simulink subsystem "WiW2025WTSubV2"  (R2024b)
settings: Solver=VariableStepAuto  StartTime=0.0  StopTime=10.0  RelTol=1e-3
values from neighbouring files (symbols this model uses):
  parWT_Init =     [parWT_Init.mat]
undefined symbols (not defined in the file or in its folder): DiscIntNeverNeededParam
settings Model: Creator=jb  LastModifiedBy=jb

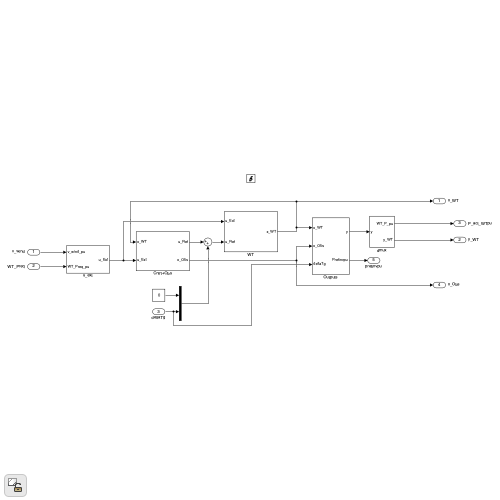
[thumbnail: Simulink's stored preview of the top-level diagram]
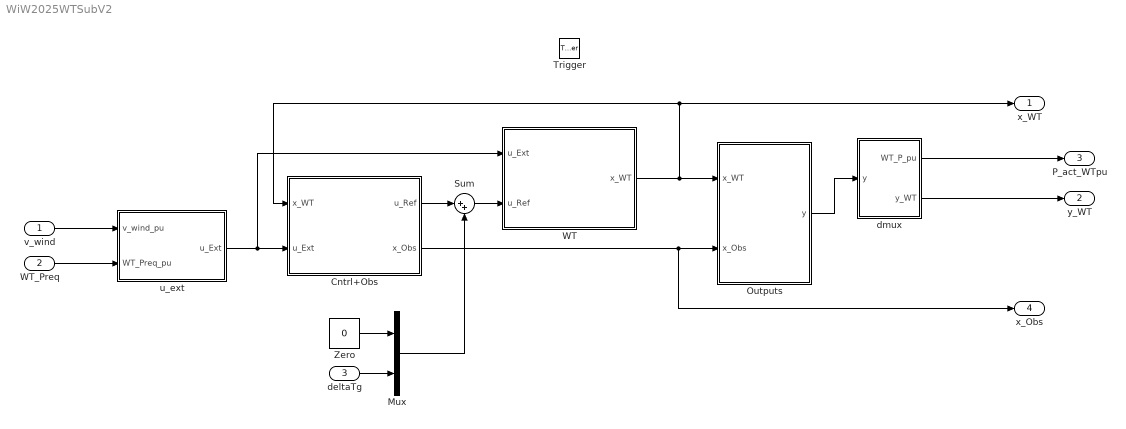
== system WiW2025WTSubV2 ==
  v_wind : Inport
  WT_Preq : Inport  Port=2
  deltaTg : Inport  Port=3
  Trigger : TriggerPort  VariantControl=(inherit)  InitialTriggerSignalState=zero
  Cntrl+Obs : Subsystem
  Mux : Mux  Inputs=2
  Outputs : Subsystem
  Sum : Sum  Inputs=|++
  WT : Subsystem
  Zero : Constant  Value=0  OutDataTypeStr=Inherit: Inherit via back propagation
  dmux : Subsystem
  u_ext : Subsystem
  x_WT : Outport
  y_WT : Outport  Port=2
  P_act_WTpu : Outport  Port=3
  x_Obs : Outport  Port=4
  wires:
  u_ext/1(u_Ext) -> Cntrl+Obs/2(u_Ext), WT/1(u_Ext)
  dmux/2(y_WT) -> y_WT/1
  WT/1(x_WT) -> Outputs/1(x_WT), Cntrl+Obs/1(x_WT), x_WT/1
  v_wind/1 -> u_ext/1(v_wind_pu)
  WT_Preq/1 -> u_ext/2(WT_Preq_pu)
  dmux/1(WT_P_pu) -> P_act_WTpu/1
  Cntrl+Obs/2(x_Obs) -> Outputs/2(x_Obs), x_Obs/1
  Outputs/1(y) -> dmux/1(y)
  Zero/1 -> Mux/1
  deltaTg/1 -> Mux/2
  Cntrl+Obs/1(u_Ref) -> Sum/1
  Sum/1 -> WT/2(u_Ref)
  Mux/1 -> Sum/2

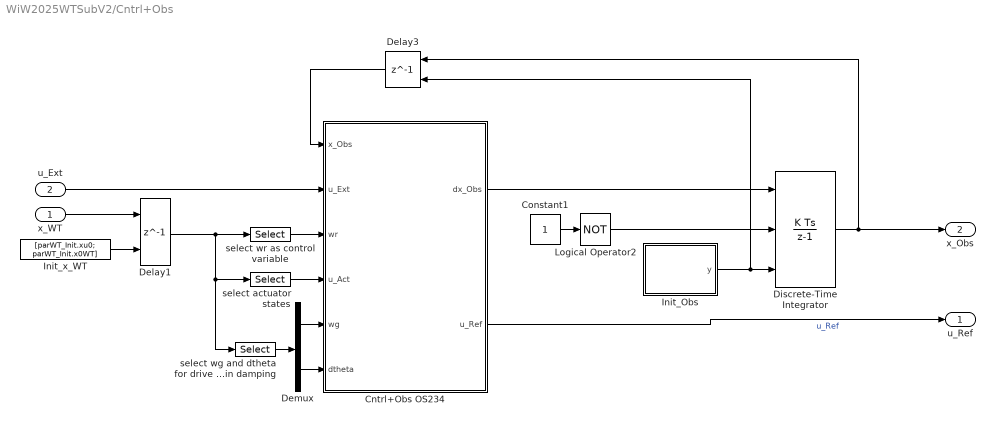
== system WiW2025WTSubV2/Cntrl+Obs ==
  x_WT : Inport  OutDataTypeStr=double  PortDimensions=11
  u_Ext : Inport  Port=2  OutDataTypeStr=double  PortDimensions=2
  Cntrl+Obs OS234 : MATLAB Function  TreatAsAtomicUnit=on
  Constant1 : Constant
  Delay1 : Delay  DelayLength=1  InitialConditionSource=Input port  InitialCondition=0
      settings: InputPortMap=u0,p4
  Delay3 : Delay  DelayLength=1  InitialConditionSource=Input port
      settings: InputPortMap=u0,p4
  Demux : Demux  Outputs=2
  Discrete-Time Integrator : DiscreteIntegrator  ExternalReset=level  InitialConditionSource=external  SampleTime=-1  ICPrevOutput=DiscIntNeverNeededParam  ICPrevScaledInput=DiscIntNeverNeededParam
  Init_Obs : MATLAB Function  TreatAsAtomicUnit=on
  Init_x_WT : Constant  Value=[parWT_Init.xu0; parWT_Init.x0WT]  VectorParams1D=off
  Logical Operator2 : Logic  Operator=NOT  AllPortsSameDT=off  OutDataTypeStr=boolean
  select actuator states : Selector  InputPortWidth=11  IndexOptions=Index vector (dialog)  Indices=[1 2]  OutputSizes=1
  select wg and dtheta for drive train damping : Selector  InputPortWidth=11  IndexOptions=Index vector (dialog)  Indices=[10,11]  OutputSizes=1
  select wr as control variable : Selector  InputPortWidth=11  IndexOptions=Index vector (dialog)  Indices=[9]  OutputSizes=1
  u_Ref : Outport  OutDataTypeStr=double  PortDimensions=2
  x_Obs : Outport  Port=2  OutDataTypeStr=double  PortDimensions=2
  wires:
  Demux/2 -> Cntrl+Obs OS234/6(dtheta)
  Demux/1 -> Cntrl+Obs OS234/5(wg)
  select wg and dtheta for drive train damping/1 -> Demux/1
  Logical Operator2/1 -> Discrete-Time Integrator/2
  Discrete-Time Integrator/1 -> x_Obs/1, Delay3/1
  Cntrl+Obs OS234/2(u_Ref) -> u_Ref/1  "u_Ref"
  select actuator states/1 -> Cntrl+Obs OS234/4(u_Act)
  Delay1/1 -> select wr as control variable/1, select actuator states/1, select wg and dtheta for drive train damping/1
  select wr as control variable/1 -> Cntrl+Obs OS234/3(wr)
  u_Ext/1 -> Cntrl+Obs OS234/2(u_Ext)
  Delay3/1 -> Cntrl+Obs OS234/1(x_Obs)
  Cntrl+Obs OS234/1(dx_Obs) -> Discrete-Time Integrator/1
  Init_x_WT/1 -> Delay1/2
  x_WT/1 -> Delay1/1
  Constant1/1 -> Logical Operator2/1
  Init_Obs/1(y) -> Delay3/2, Discrete-Time Integrator/3

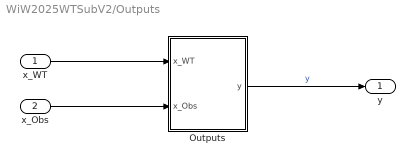
== system WiW2025WTSubV2/Outputs ==
  x_WT : Inport  OutDataTypeStr=double  PortDimensions=11
  x_Obs : Inport  Port=2  OutDataTypeStr=double  PortDimensions=2
  Outputs : MATLAB Function  TreatAsAtomicUnit=on
  y : Outport  OutDataTypeStr=double  PortDimensions=14
  wires:
  Outputs/1(y) -> y/1  "y"
  x_Obs/1 -> Outputs/2(x_Obs)
  x_WT/1 -> Outputs/1(x_WT)

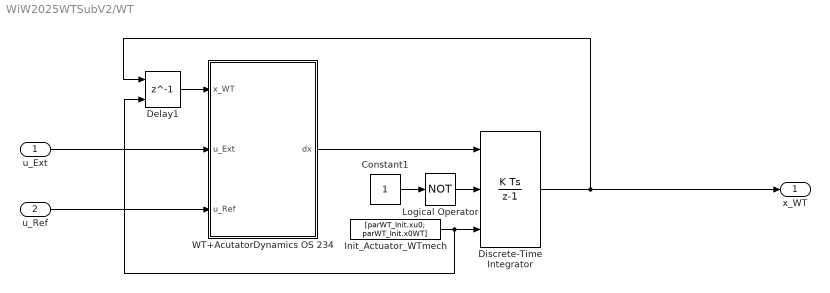
== system WiW2025WTSubV2/WT ==
  u_Ext : Inport  OutDataTypeStr=double  PortDimensions=2
  u_Ref : Inport  Port=2  OutDataTypeStr=double  PortDimensions=2
  Constant1 : Constant
  Delay1 : Delay  DelayLength=1  InitialConditionSource=Input port
      settings: InputPortMap=u0,p4
  Discrete-Time Integrator : DiscreteIntegrator  ExternalReset=level  InitialConditionSource=external  SampleTime=-1  ICPrevOutput=DiscIntNeverNeededParam  ICPrevScaledInput=DiscIntNeverNeededParam
  Init_Actuator_WTmech : Constant  Value=[parWT_Init.xu0; parWT_Init.x0WT]  VectorParams1D=off
  Logical Operator : Logic  Operator=NOT  AllPortsSameDT=off  OutDataTypeStr=boolean
  WT+AcutatorDynamics OS 234 : MATLAB Function  TreatAsAtomicUnit=on
  x_WT : Outport  OutDataTypeStr=double  PortDimensions=11
  wires:
  u_Ext/1 -> WT+AcutatorDynamics OS 234/2(u_Ext)
  Logical Operator/1 -> Discrete-Time Integrator/2
  Constant1/1 -> Logical Operator/1
  Init_Actuator_WTmech/1 -> Discrete-Time Integrator/3, Delay1/2
  u_Ref/1 -> WT+AcutatorDynamics OS 234/3(u_Ref)
  WT+AcutatorDynamics OS 234/1(dx) -> Discrete-Time Integrator/1
  Discrete-Time Integrator/1 -> x_WT/1, Delay1/1
  Delay1/1 -> WT+AcutatorDynamics OS 234/1(x_WT)

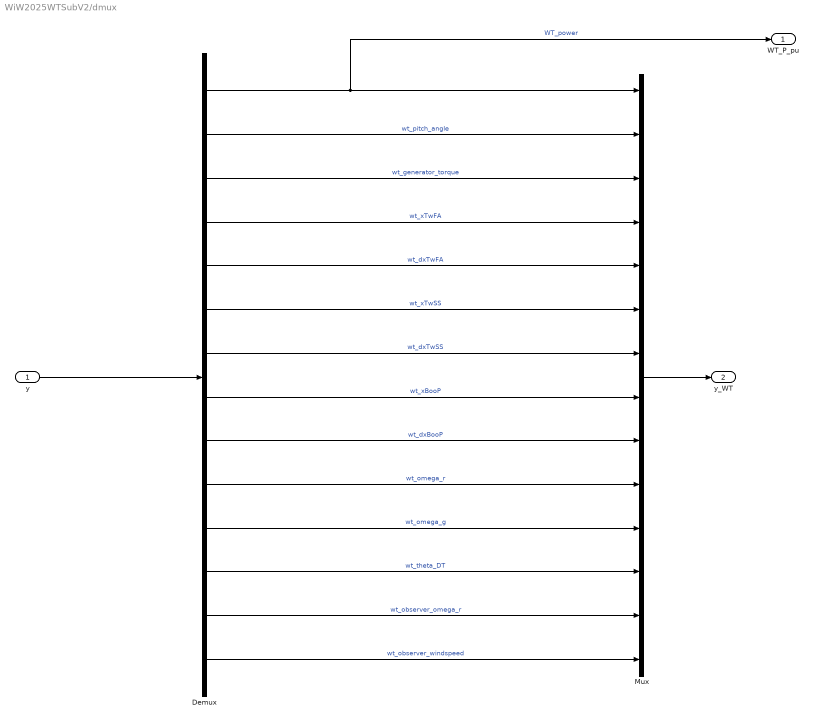
== system WiW2025WTSubV2/dmux ==
  y : Inport  OutDataTypeStr=double  PortDimensions=14
  Demux : Demux  Outputs=14
  Mux : Mux  Inputs=14
  WT_P_pu : Outport  OutDataTypeStr=double  PortDimensions=1
  y_WT : Outport  Port=2  OutDataTypeStr=double  PortDimensions=14
  wires:
  Demux/8 -> Mux/8  "wt_xBooP"
  Demux/5 -> Mux/5  "wt_dxTwFA"
  Demux/9 -> Mux/9  "wt_dxBooP"
  Demux/11 -> Mux/11  "wt_omega_g"
  Demux/12 -> Mux/12  "wt_theta_DT"
  Demux/1 -> WT_P_pu/1, Mux/1  "WT_power"
  Demux/7 -> Mux/7  "wt_dxTwSS"
  Demux/6 -> Mux/6  "wt_xTwSS"
  y/1 -> Demux/1
  Demux/3 -> Mux/3  "wt_generator_torque"
  Demux/14 -> Mux/14  "wt_observer_windspeed"
  Demux/10 -> Mux/10  "wt_omega_r"
  Demux/4 -> Mux/4  "wt_xTwFA"
  Demux/13 -> Mux/13  "wt_observer_omega_r"
  Demux/2 -> Mux/2  "wt_pitch_angle"
  Mux/1 -> y_WT/1

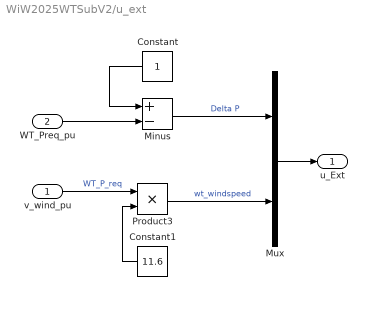
== system WiW2025WTSubV2/u_ext ==
  v_wind_pu : Inport
  WT_Preq_pu : Inport  Port=2
  Constant : Constant
  Constant1 : Constant  Value=11.6
  Minus : Sum  Inputs=+-
  Mux : Mux  Inputs=2
  Product3 : Product
  u_Ext : Outport
  wires:
  v_wind_pu/1 -> Product3/1  "WT_P_req"
  WT_Preq_pu/1 -> Minus/2
  Mux/1 -> u_Ext/1
  Product3/1 -> Mux/2  "wt_windspeed"
  Constant/1 -> Minus/1
  Minus/1 -> Mux/1  "Delta P"
  Constant1/1 -> Product3/2

== matlab function WiW2025WTSubV2/Cntrl+Obs/Cntrl+Obs OS234 ==
  data: dx_Obs output size=2; x_Obs input size=2; u_Ext input size=2; wr input; u_Act input; wg input; dtheta input; u_Ref output size=2; parWT parameter
function [dx_Obs,u_Ref] = mdlDerivatives(x_Obs,u_Ext,wr,u_Act,wg,dtheta,parWT)

%% THIS IS FOR OS 2,3,4,5 ONLY!!!!

%% Calculate Controller Inputs for Wind turbine and calulate Observer states

% x_obs = [wr_obs; v_obs]                Observer States 
% u_Act = [beata_actual; Tg_actual]   Current pitch angle and generator torque
% u_Ext = [dP; v]                   v: Wind speed and dP: relative power setpoint
%

% -----------------------------------------------------
%                   Basic definitios
% -----------------------------------------------------

par = parWT.CTRL; % Turbine Info Struct

P_req_rel = u_Ext(1); 
windspeed = u_Ext(2);

% x_obs = [wr_obs v_obs]
xx = x_Obs; %  observer States 


% define premise variables
% switch par.WTversion
%     case {0,5}
%         % premise vector  [OS ,v , dp]
%         z = [par.OS windspeed P_req_rel];
%     case {1,2,3,4}
%         % premise vector  [v , dp]
        z = [windspeed P_req_rel];
% end


% switch par.WTversion
%     case 5
%         z(2) = xx(end);
%     otherwise 
%         % -> Sieht so aus als würde hier die premise variable auf den letzten State
%         % des Zustandsvektors gestzt -> könnte die windgeschwindigkeit aus
%         % observer sein?
        z(1) = xx(end); % Premise variable -> observer windspeed
% end



% Membership Functions for PDC Controller
hk = calc_TriangMemFcn(z,par.TSmdl.LinPoints_c.z1,par.TSmdl.LinPoints_c.z2);
hl = hk;

u = zeros(size(par.TSmdl.LTI(1).u0));

% calculate derivatives
dxx = zeros(size(xx)); % oserver states


% -----------------------------------------------------
%              Controller Input Calculations (PDC)
% -----------------------------------------------------
%
% Based on Parallel Distributed Compensation Controller desing (PDC)
% u = - hk(z) Kk * x
% Calculate Inputs u based on Membership Functions hk of all submodels
% The controller only takes x = wr (rotor speed) as control variabel

for k = 1:1:length(hk)
     % if par.WTversion == 2 || par.WTversion == 3 || par.WTversion == 4 || par.WTversion == 5
         % Here the control variable is the rotor speed wr
         Kk = par.TSmdl.LTI_c(k).K;
         x0k = par.TSmdl.LTI_c(k).x0(1);
         u0k = par.TSmdl.LTI_c(k).u0;

    u = u + hk(k)*(-Kk*(x_Obs(1)-x0k)+u0k); % xx(n+1:end-1) -> wr_obs as control variabel n+1=10 
    if u(1) < 0 % If pitch angle < 0 is demanded set it to zero
        u(1) = 0;
    end
end

% -----------------------------------------------------
%                      Observer
% -----------------------------------------------------
% Sieht nach Observer aus was hier passiert
% Calculate observer error e -> [wr;windspeed]-[wr_obs,windspeed_obs]
e = [wr;windspeed]-x_Obs; 

Aol     = 0;
Bol     = 0;
Lol     = 0;
Co      = 0;
xo0l    = 0;
u0l     = 0;
l       = 0;


for l =1:length(hl)
    Aol = par.TSmdl.LTI_c(l).A; % 2x2 Matrix
    Bol = par.TSmdl.LTI_c(l).B; % 2x2 Matrix
    Lol = par.TSmdl.LTI_c(l).L; % 2x1 Vector
    Co = par.TSmdl.LTI_c(l).C; % 1x2 Vector
    xo0l = par.TSmdl.LTI_c(l).x0;
    u0l = par.TSmdl.LTI_c(l).u0;
    % Observer State Transitions get added seperately here -> dxx(n+1:end)
    dxx(1:2) = dxx(1:2) + ...
        hl(l)*( Aol*(xx-xo0l) + Bol*(u_Act-u0l) + Lol*Co*e);
end


% -----------------------------------------------------
%                   Final Output
% -----------------------------------------------------
u_Ref = u;
dx_Obs = dxx;

end

function[h] = calc_TriangMemFcn(z,LinPointsWind,LinPointsPRM)
% calculate weighting functions
wv = zeros(numel(LinPointsWind),1);
wPRM = zeros(numel(LinPointsPRM),1);

for idim = 1 : 2
    switch idim
        case 1
            lps = LinPointsWind;
            if z(idim) <= lps(1)
                wv(1) = 1;
            else
                for iLP = 2 : numel(lps)
                    if z(idim) < lps(iLP)
                        wv(iLP-1) = 1-(z(idim)-lps(iLP-1))/(lps(iLP)-lps(iLP-1));
                        wv(iLP) = (z(idim)-lps(iLP-1))/(lps(iLP)-lps(iLP-1));
                        break
                    end
                    if z(idim) >= lps(numel(lps))
                        wv(numel(lps)) = 1;
                    end
                end
            end
        case 2
            lps = LinPointsPRM;
            if z(idim) <= lps(1)
                wPRM(1) = 1;
            else
                for iLP = 2 : numel(lps)
                    if z(idim) < lps(iLP)
                        wPRM(iLP-1) = 1-(z(idim)-lps(iLP-1))/(lps(iLP)-lps(iLP-1));
                        wPRM(iLP) = (z(idim)-lps(iLP-1))/(lps(iLP)-lps(iLP-1));
                        break
                    end
                    if z(idim) >= lps(numel(lps))
                        wPRM(numel(lps)) = 1;
                    end
                end
            end
    end
end
h = wv*wPRM';
h = h';
h = h(:);    


end

== matlab function WiW2025WTSubV2/Cntrl+Obs/Init_Obs ==
  data: y output; parWT_Init parameter
function y = fcn(parWT_Init)

y = parWT_Init.x0obs';

== matlab function WiW2025WTSubV2/Outputs/Outputs ==
  data: x_WT input size=11; x_Obs input; y output size=14; parWT parameter
function y  = mdlOutputs(x_WT, x_Obs, parWT)

par = parWT;
x = [x_WT; x_Obs];

xu = x(1:2); 
x = x(3:end); 

pmax_global = par.WT.TSmdl.LTI(end-numel(par.WT.TSmdl.deltaP)+1).u0(2)*par.WT.TSmdl.LTI(end-numel(par.WT.TSmdl.deltaP)+1).x0(8);
P_sub_abs = x(8)*xu(2)/pmax_global;

y = [ P_sub_abs; xu; x];



end

== matlab function WiW2025WTSubV2/WT/WT+AcutatorDynamics OS 234 ==
  data: x_WT input size=11; u_Ext input size=2; u_Ref input; dx output size=11; parWT parameter
function dx = mdlDerivatives(x_WT, u_Ext, u_Ref, parWT)

%% THIS IS FOR OS 1,2,3,4 ONLY!!!!

%% Calculate State Transitions based on TS mdl
    % dx = hi*(Ai x + Bi u + Bdi w)
    % x = [beta Tg | x_TwFA dx_TwFA x_TwSS dx_TwSS x_BooP dx_BooP wr wg theta_DT]
    % u_ref WT -> Inputs [beta_d_ref, Tg_ref] (Pitchangle Torque_Generator)
    % w -> Disturbance (Windspeed)
    %
    % Full State Vector of System with all additions (Actuator Dynamics, WT States, Observer
    % States)
    % xx -> [beta Tg | x_TwFA dx_TwFA x_TwSS dx_TwSS x_BooP dx_BooP wr wg theta_DT]
    
% ! The System gets augmented with Actuator dynamics such that the final
% State Vector becomes

% Current Setup: The Membership functions for the States of the Turbine get
% calculated with the real windspeed. The Membership functions of the
% Controller get calculated with the observed windspeed

% Parameterization through par_WT struct
% Function Inputs u -> [dP, vWind] (Power setpoint, windspeed) 
% Actuator Inputs u -> [beta_d, Tg] (Pitchangle, Torque_Generator)

% -----------------------------------------------------
%                   Basic definitios
% -----------------------------------------------------

par = parWT; % Turbine Info Struct

P_req_rel = u_Ext(1); 
windspeed = u_Ext(2);

% xu = [beta Tg]^T
xu = x_WT(1:2); % states for the actuator dynamics

% xx [x_TwFA dx_TwFA x_TwSS dx_TwSS x_BooP dx_BooP wr wg theta_DT]^T
xx = x_WT(3:end); % state of the Turbine movement


% -----------------------------------------------------
%                Define premise variable
% -----------------------------------------------------

%switch par.WTversion
%    case {0,5}
        % premise vector  [OS ,v , dp]
%        z = [par.OS windspeed P_req_rel];
%    case {1,2,3,4}
        % premise vector  [v , dp]
        z = [windspeed P_req_rel];
%end

% -----------------------------------------------------
%                    calculate membership
% -----------------------------------------------------
% -> needs to be the real windpeed
% Membership functions for i
hi = calc_TriangMemFcn(z,par.WT.TSmdl.LinPoints.z1,par.WT.TSmdl.LinPoints.z2); % with true wind from data

% -----------------------------------------------------
%                    Actuator Dynamics
% -----------------------------------------------------
tauPitchR = parWT.WT.tauPitchR;
tauTg = parWT.WT.tauTg;

% u -> Inputs [beta_d, Tg]
dxu     = zeros(2,1); 
%dxu(1)  = -1/.1*xu(1) + 1/.1*u_Ref(1);
dxu(1)  = -1/tauPitchR*xu(1) + 1/tauPitchR*u_Ref(1);
dxu(2)  = -1/tauTg*xu(2) + 1/tauTg*u_Ref(2);

% write current actuator state to input
uWT = zeros(size(par.WT.TSmdl.LTI(1).u0));
uWT = xu; 

% -----------------------------------------------------
%                    State Transition
% -----------------------------------------------------

% Calculate State Transitions based on TS mdl
% dx = hi*(Ai x + Bi u + Bdi w)
% x -> States [x_TwFA dx_TwFA x_TwSS dx_TwSS x_BooP dx_BooP wr wg theta_DT]
% u -> Inputs [beta_d, Tg] (Pitchangle Torque_Generator)
% w -> Disturbance (Windspeed)

Ai      = 0;
Bi      = 0;
x0i     = 0;
u0i     = 0;
Bdi     = 0;
d0i     = 0;
i       = 0;

% calculate derivatives
dxx = zeros(size(xx)); % states + recons. states + augmented wind state v
n = length(par.WT.TSmdl.LTI(1).x0); % Number of States of System (here 9 States)


for i = 1:length(hi)
    Ai = par.WT.TSmdl.LTI(i).A; % 9x9 Matrix
    Bi = par.WT.TSmdl.LTI(i).B; % 9x2 Matrix
    x0i = par.WT.TSmdl.LTI(i).x0;
    u0i = par.WT.TSmdl.LTI(i).u0; 
    Bdi = par.WT.TSmdl.LTI(i).Bd; 
    d0i = par.WT.TSmdl.LTI(i).d0;

    % Here only the Actuator Dynamics and Turbine States get calculated 
    dxx(1:n) = dxx(1:n) + hi(i)*( Ai*(xx-x0i) + Bi*(uWT-u0i) + Bdi*(windspeed-d0i));
end



% -----------------------------------------------------
%                   Final Output
% -----------------------------------------------------

dx = [dxu ; dxx]; 


end

function[h] = calc_TriangMemFcn(z,LinPointsWind,LinPointsPRM)
% calculate weighting functions
wv = zeros(numel(LinPointsWind),1);
wPRM = zeros(numel(LinPointsPRM),1);

for idim = 1 : 2
    switch idim
        case 1
            lps = LinPointsWind;
            if z(idim) <= lps(1)
                wv(1) = 1;
            else
                for iLP = 2 : numel(lps)
                    if z(idim) < lps(iLP)
                        wv(iLP-1) = 1-(z(idim)-lps(iLP-1))/(lps(iLP)-lps(iLP-1));
                        wv(iLP) = (z(idim)-lps(iLP-1))/(lps(iLP)-lps(iLP-1));
                        break
                    end
                    if z(idim) >= lps(numel(lps))
                        wv(numel(lps)) = 1;
                    end
                end
            end
        case 2
            lps = LinPointsPRM;
            if z(idim) <= lps(1)
                wPRM(1) = 1;
            else
                for iLP = 2 : numel(lps)
                    if z(idim) < lps(iLP)
                        wPRM(iLP-1) = 1-(z(idim)-lps(iLP-1))/(lps(iLP)-lps(iLP-1));
                        wPRM(iLP) = (z(idim)-lps(iLP-1))/(lps(iLP)-lps(iLP-1));
                        break
                    end
                    if z(idim) >= lps(numel(lps))
                        wPRM(numel(lps)) = 1;
                    end
                end
            end
    end
end
h = wv*wPRM';
h = h';
h = h(:);    


end
